simulink model "Velocity_Expanded_Model"  (R2018b)
settings: Solver=VariableStepAuto  StartTime=0.0  StopTime=120  RelTol=1e-3
model workspace (MAT data in the model file):
  A = Simulink.Parameter
  A.Value = 2.4
  A.DataType = 'auto'
  A.DocUnits = '<m*2>'
  A.Dimensions = [1 1]
  B = Simulink.Parameter
  B.Value = 0.4
  B.DataType = 'auto'
  B.Dimensions = [1 1]
  Cd = Simulink.Parameter
  Cd.Value = 0.32
  Cd.DataType = 'auto'
  Cd.Dimensions = [1 1]
  Cr = Simulink.Parameter
  Cr.Value = 0.1
  Cr.DataType = 'auto'
  Cr.Dimensions = [1 1]
  Tm = Simulink.Parameter
  Tm.Value = 190
  Tm.DataType = 'auto'
  Tm.Dimensions = [1 1]
  g = Simulink.Parameter
  g.Value = 9.8
  g.DataType = 'auto'
  g.DocUnits = '<N>'
  g.Dimensions = [1 1]
  wm = Simulink.Parameter
  wm.Value = 420
  wm.DataType = 'auto'
  wm.Dimensions = [1 1]
undefined symbols (not defined in the file): an, b, m, W, Wm
settings Model: Creator=Kacpix  LastModifiedBy=Kacpix

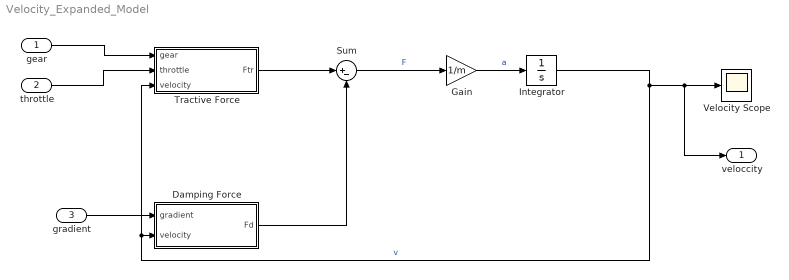
== system Velocity_Expanded_Model ==
  "gear " : Inport
  "throttle " : Inport  Port=2
  "gradient " : Inport  Port=3
  "Damping Force " : Subsystem
  Gain : Gain  Gain=1/m
  Integrator : Integrator
  Sum : Sum  Inputs=|+-
  Tractive Force : Subsystem
  Velocity Scope : Scope
  "veloccity " : Outport
  wires:
  Integrator/1 -> Tractive Force/3(velocity), "Damping Force "/2("velocity "), "veloccity "/1, Velocity Scope/1  "v"
  Gain/1 -> Integrator/1  "a"
  Sum/1 -> Gain/1  "F"
  "gradient "/1 -> "Damping Force "/1("gradient ")
  "Damping Force "/1("Fd ") -> Sum/2
  Tractive Force/1("Ftr ") -> Sum/1
  "throttle "/1 -> Tractive Force/2(throttle)
  "gear "/1 -> Tractive Force/1(gear)

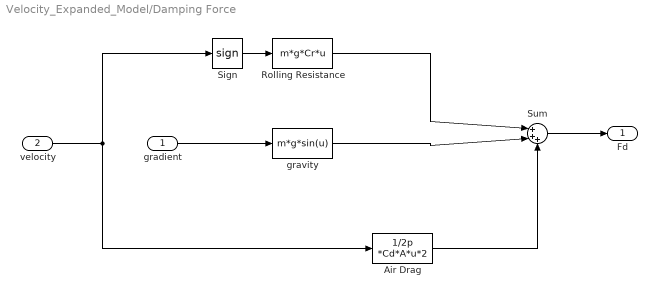
== system Velocity_Expanded_Model/Damping Force  ==
  "gradient " : Inport
  "velocity " : Inport  Port=2
  "Air Drag " : Fcn  Expr=1/2p *Cd*A*u*2
  "Rolling Resistance " : Fcn  Expr=m*g*Cr*u
  Sign : Signum
  Sum : Sum  Inputs=|+++
  gravity : Fcn  Expr=m*g*sin(u)
  "Fd " : Outport
  wires:
  "velocity "/1 -> "Air Drag "/1, Sign/1
  Sign/1 -> "Rolling Resistance "/1
  Sum/1 -> "Fd "/1
  "Rolling Resistance "/1 -> Sum/1
  "gradient "/1 -> gravity/1
  gravity/1 -> Sum/2
  "Air Drag "/1 -> Sum/3

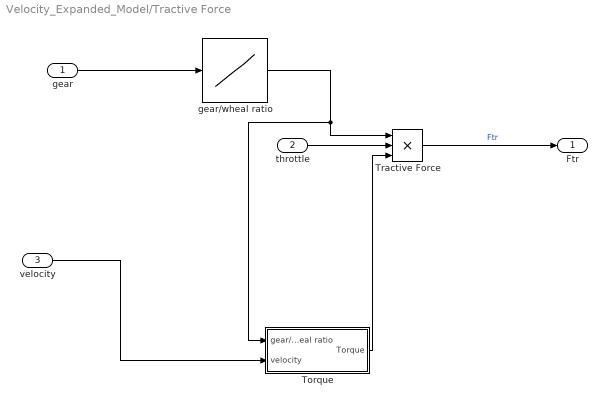
== system Velocity_Expanded_Model/Tractive Force ==
  gear : Inport
  throttle : Inport  Port=2
  velocity : Inport  Port=3
  "Torque " : Subsystem
  "Tractive Force " : Product  Inputs=3
  "gear/wheal ratio " : Lookup_n-D  NumberOfTableDimensions=1  BreakpointsForDimension1=[1:5]  Table=int16([40,25,15,12,10])  InternalRulePriority=Speed  RndMeth=Simplest  InputSameDT=on
  "Ftr " : Outport
  wires:
  "Tractive Force "/1 -> "Ftr "/1  "Ftr"
  gear/1 -> "gear/wheal ratio "/1
  "gear/wheal ratio "/1 -> "Tractive Force "/1, "Torque "/1("gear/wheal ratio ")
  throttle/1 -> "Tractive Force "/2
  velocity/1 -> "Torque "/2("velocity ")
  "Torque "/1("Torque ") -> "Tractive Force "/3

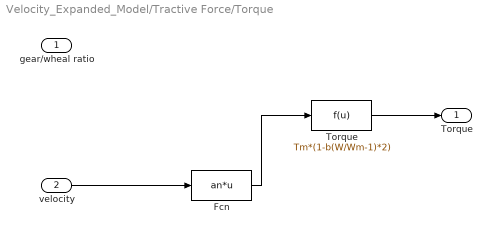
== system Velocity_Expanded_Model/Tractive Force/Torque  ==
  "gear/wheal ratio " : Inport
  "velocity " : Inport  Port=2
  Fcn : Fcn  Expr=an*u
  Torque : Fcn  Expr=Tm*(1-b(W/Wm-1)*2)
  "Torque " : Outport
  wires:
  Fcn/1 -> Torque/1
  "velocity "/1 -> Fcn/1
  Torque/1 -> "Torque "/1
